simulink model "dspStartModel_fft"  (Simulink 7.4)
settings: Solver=VariableStepDiscrete  StartTime=0  StopTime=1000  RelTol=1e-3
undefined symbols (not defined in the file or in its folder): referenceDSP
libraries: dspbuff3 x7, dspsigattribs x4, dspxfrm3 x4, dspindex x4
settings Model: Creator=Administrator  LastModifiedBy=Administrator
settings SimEventsCC: propDiagAttribOutput=1  propDiagFcnCallOutput=1  propDiagStatOutput=0

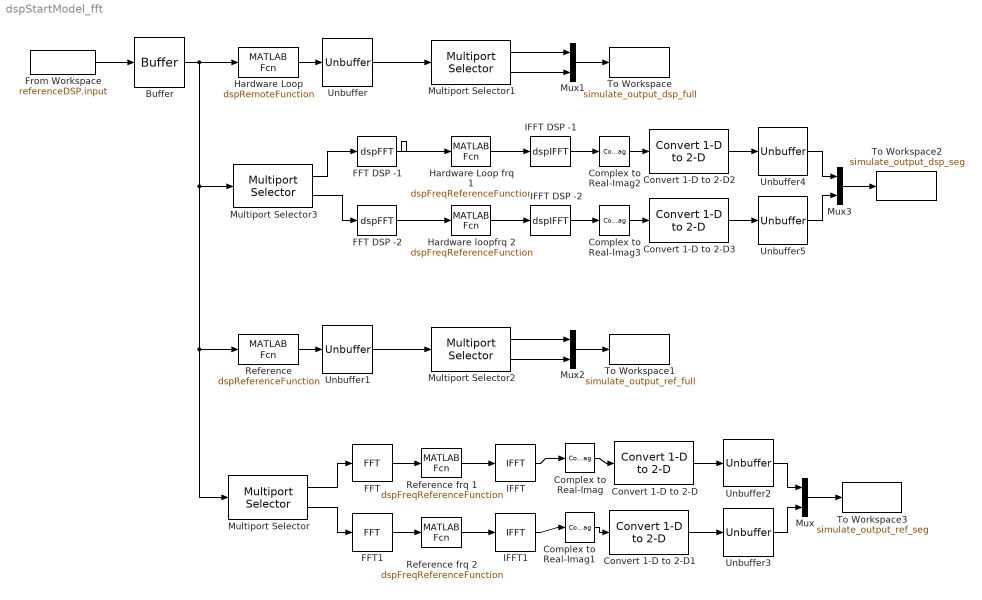
== system dspStartModel_fft ==
  Buffer : dspbuff3/Buffer  N=referenceDSP.dspCfg.buffersize  V=0  ic=0
  Complex to Real-Imag{,1..3} (4 alike) : ComplexToRealImag  Output=Real
  Convert 1-D to 2-D{,1..3} (4 alike) : dspsigattribs/Convert 1-D to 2-D  SystemSampleTime=-1  M=referenceDSP.dspCfg.buffersize  N=1  frameBasedOut=on
  FFT : dspxfrm3/FFT  DialogController=dspDDGCreate  DialogControllerArgs=DataTag0  CompMethod=Table lookup  TableOpt=NEW  TableOptActive=Speed  BitRevOrder=off  InheritFFTLength=on  FFTLength=64  SkipNorm=off  roundingMode=Floor  overflowMode=off
  FFT DSP -1 : MATLABFcn  MATLABFcn=dspFFT  OutputSignalType=complex  Output1D=off
  FFT DSP -2 : MATLABFcn  MATLABFcn=dspFFT  OutputSignalType=complex  Output1D=off
  FFT1 : dspxfrm3/FFT  DialogController=dspDDGCreate  DialogControllerArgs=DataTag1  CompMethod=Table lookup  TableOpt=NEW  TableOptActive=Speed  BitRevOrder=off  InheritFFTLength=on  FFTLength=64  SkipNorm=off  roundingMode=Floor  overflowMode=off
  From Workspace : FromWorkspace  VariableName=referenceDSP.input  SampleTime=1
  Hardware Loop : MATLABFcn  MATLABFcn=dspRemoteFunction  Output1D=off
  Hardware Loop frq 1 : MATLABFcn  MATLABFcn=dspFreqReferenceFunction  OutputSignalType=complex  Output1D=off
  Hardware loopfrq 2 : MATLABFcn  MATLABFcn=dspFreqReferenceFunction  OutputSignalType=complex  Output1D=off
  IFFT : dspxfrm3/IFFT  DialogController=dspDDGCreate  DialogControllerArgs=DataTag2  CompMethod=Table lookup  TableOpt=NEW  TableOptActive=Speed  BitRevOrder=off  cs_in=off  SkipNorm=on  InheritFFTLength=on  FFTLength=64  mode=Complex  outSamplingMode=Sample based  roundingMode=Floor  overflowMode=off
  IFFT DSP -1 : MATLABFcn  MATLABFcn=dspIFFT  Output1D=off
  IFFT DSP -2 : MATLABFcn  MATLABFcn=dspIFFT  Output1D=off
  IFFT1 : dspxfrm3/IFFT  DialogController=dspDDGCreate  DialogControllerArgs=DataTag3  CompMethod=Table lookup  TableOpt=NEW  TableOptActive=Speed  BitRevOrder=off  cs_in=off  SkipNorm=on  InheritFFTLength=on  FFTLength=64  mode=Complex  outSamplingMode=Sample based  roundingMode=Floor  overflowMode=off
  Multiport Selector{,1..3} (4 alike) : dspindex/Multiport Selector  rowsOrCols=Columns  idxCellArray={ 1, 2 }  idxErrMode=Clip Index
  Mux{,1..3} (4 alike) : Mux  Inputs=2
  Reference : MATLABFcn  MATLABFcn=dspReferenceFunction  Output1D=off
  Reference frq 1 : MATLABFcn  MATLABFcn=dspFreqReferenceFunction  OutputSignalType=complex  Output1D=off
  Reference frq 2 : MATLABFcn  MATLABFcn=dspFreqReferenceFunction  OutputSignalType=complex  Output1D=off
  To Workspace : ToWorkspace  VariableName=simulate_output_dsp_full  SampleTime=-1  SaveFormat=Structure
  To Workspace1 : ToWorkspace  VariableName=simulate_output_ref_full  SampleTime=-1  SaveFormat=Structure
  To Workspace2 : ToWorkspace  VariableName=simulate_output_dsp_seg  SampleTime=-1  SaveFormat=Structure
  To Workspace3 : ToWorkspace  VariableName=simulate_output_ref_seg  SampleTime=-1  SaveFormat=Structure
  Unbuffer{,1..5} (6 alike) : dspbuff3/Unbuffer  ic=0
  wires:
  From Workspace/1 -> Buffer/1
  Buffer/1 -> Hardware Loop/1, Multiport Selector3/1, Reference/1, Multiport Selector/1
  Hardware Loop/1 -> Unbuffer/1
  Unbuffer1/1 -> Multiport Selector2/1
  Reference/1 -> Unbuffer1/1
  Multiport Selector/1 -> FFT/1
  Multiport Selector/2 -> FFT1/1
  Mux/1 -> To Workspace3/1
  Unbuffer/1 -> Multiport Selector1/1
  Multiport Selector1/1 -> Mux1/1
  Multiport Selector1/2 -> Mux1/2
  Mux1/1 -> To Workspace/1
  Multiport Selector2/1 -> Mux2/1
  Multiport Selector2/2 -> Mux2/2
  Mux2/1 -> To Workspace1/1
  FFT/1 -> Reference frq 1/1
  FFT1/1 -> Reference frq 2/1
  IFFT1/1 -> Complex to Real-Imag1/1
  Convert 1-D to 2-D/1 -> Unbuffer2/1
  Convert 1-D to 2-D1/1 -> Unbuffer3/1
  Unbuffer2/1 -> Mux/1
  IFFT/1 -> Complex to Real-Imag/1
  Unbuffer3/1 -> Mux/2
  Multiport Selector3/2 -> FFT DSP -2/1
  Mux3/1 -> To Workspace2/1
  IFFT DSP -2/1 -> Complex to Real-Imag3/1
  Convert 1-D to 2-D2/1 -> Unbuffer4/1
  Convert 1-D to 2-D3/1 -> Unbuffer5/1
  Unbuffer4/1 -> Mux3/1
  IFFT DSP -1/1 -> Complex to Real-Imag2/1
  Complex to Real-Imag2/1 -> Convert 1-D to 2-D2/1
  Unbuffer5/1 -> Mux3/2
  Complex to Real-Imag3/1 -> Convert 1-D to 2-D3/1
  FFT DSP -2/1 -> Hardware loopfrq 2/1
  FFT DSP -1/1 -> Hardware Loop frq 1/1
  Multiport Selector3/1 -> FFT DSP -1/1
  Complex to Real-Imag/1 -> Convert 1-D to 2-D/1
  Complex to Real-Imag1/1 -> Convert 1-D to 2-D1/1
  Hardware Loop frq 1/1 -> IFFT DSP -1/1
  Hardware loopfrq 2/1 -> IFFT DSP -2/1
  Reference frq 1/1 -> IFFT/1
  Reference frq 2/1 -> IFFT1/1
